simulink model "BE_simu5"  (R2018b)
settings: Solver=VariableStepAuto  StartTime=0.0  StopTime=100  RelTol=1e-3
values from neighbouring files (symbols this model uses):
  assist = 2    [BE_eletr.m]
  lambm = 0.0744    [BE_eletr.m]
  Ls = 0.0021    [BE_eletr.m]
  Np = 52    [BE_eletr.m]
  Rs = 0.124    [BE_eletr.m]
  s = 0.07    [BE_eletr.m]
libraries: simulink x2
settings Model: Creator=antoi  LastModifiedBy=piffercg
settings SolverCC: AlgebraicLoopSolver=LineSearch
settings DataIOCC: ReturnWorkspaceOutputs=on

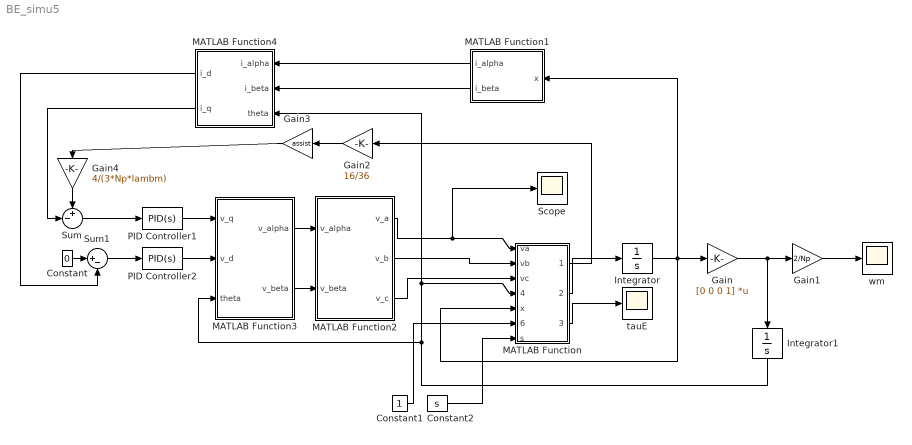
== system BE_simu5 ==
  Constant : Constant  Value=0
  Constant1 : Constant
  Constant2 : Constant  Value=s
  Gain : Gain  Gain=[0 0 0 1]  Multiplication=Matrix(K*u)
  Gain1 : Gain  Gain=2/Np
  Gain2 : Gain  Gain=16/36
  Gain3 : Gain  Gain=assist
  Gain4 : Gain  Gain=4/(3*Np*lambm)
  Integrator : Integrator  InitialCondition=[0 ;0 ;0;0]
  Integrator1 : Integrator
  MATLAB Function : MATLAB Function  TreatAsAtomicUnit=on
  MATLAB Function1 : MATLAB Function  TreatAsAtomicUnit=on
  MATLAB Function2 : MATLAB Function  TreatAsAtomicUnit=on
  MATLAB Function3 : MATLAB Function  TreatAsAtomicUnit=on
  MATLAB Function4 : MATLAB Function  TreatAsAtomicUnit=on
  PID Controller1 : simulink/Continuous/PID Controller  Controller=PID  Form=Parallel  TimeDomain=Continuous-time  SampleTime=-1  IntegratorMethod=Forward Euler  FilterMethod=Forward Euler  ControllerParametersSource=internal  P=Rs  I=Rs*Rs/Ls  D=0  UseFilter=on  N=100  TunerSelectOption=Transfer Function Based (PID Tuner App)  InitialConditionSource=internal  InitialConditionForIntegrator=0  InitialConditionForFilter=0  DifferentiatorICPrevScaledInput=0  ExternalReset=none  TrackingMode=off  Kt=1  LimitOutput=off  UpperSaturationLimit=inf  LowerSaturationLimit=-inf  LinearizeAsGain=on  AntiWindupMode=none  Kb=1  POutMin=[]  POutMax=[]  IOutMin=[]  IOutMax=[]  DOutMin=[]  DOutMax=[]  NOutMin=[]  NOutMax=[]  SumOutMin=[]  SumOutMax=[]  SaturationOutMin=[]  SaturationOutMax=[]  PParamMin=[]  PParamMax=[]  IParamMin=[]  IParamMax=[]  DParamMin=[]  DParamMax=[]  NParamMin=[]  NParamMax=[]  KbParamMin=[]  KbParamMax=[]  KtParamMin=[]  KtParamMax=[]  KbOutMin=[]  KbOutMax=[]  KtOutMin=[]  KtOutMax=[]  IntegratorOutMin=[]  IntegratorOutMax=[]  FilterOutMin=[]  FilterOutMax=[]  SumI1OutMin=[]  SumI1OutMax=[]  SumI2OutMin=[]  SumI2OutMax=[]  SumI3OutMin=[]  SumI3OutMax=[]  SumI4OutMin=[]  SumI4OutMax=[]  SumDOutMin=[]  SumDOutMax=[]  DifferentiatorOutMin=[]  DifferentiatorOutMax=[]  FilterDiffOutCoefMin=[]  FilterDiffOutCoefMax=[]  ReciprocalOutMin=[]  ReciprocalOutMax=[]  SumDenOutMin=[]  SumDenOutMax=[]  SumNumOutMin=[]  SumNumOutMax=[]  DivideOutMin=[]  DivideOutMax=[]  IntegratorContinuousStateAttributes=''  IntegratorStateMustResolveToSignalObject=off  IntegratorRTWStateStorageClass=Auto  FilterContinuousStateAttributes=''  FilterStateMustResolveToSignalObject=off  FilterRTWStateStorageClass=Auto  ParallelPVariant=InternalParameters  IdealPVariant=Disabled  IVariant=InternalParameters  DVariant=InternalParameters  IntegratorVariant=Continuous  SatVariant=Disabled  AWVariant=Passthrough  PCopyVariant=Disabled  TRVariant=Disabled  FdbkBlocksVariant=Forward  IdealPFdbkVariant=Disabled  SatFdbkVariant=Disabled  DerivativeFilterVariant=ContFilter  NVariant=InternalParameters  NCopyVariant=Disabled  FilterICVariant=InternalICsFilter  IntegratorICVariant=InternalICs  ExternalResetVariant=Disabled  TRSumVariant=Passthrough  SumFdbkVariant=Disabled  SumVariant=Sum_PID
  PID Controller2 : simulink/Continuous/PID Controller  Controller=PID  Form=Parallel  TimeDomain=Continuous-time  SampleTime=-1  IntegratorMethod=Forward Euler  FilterMethod=Forward Euler  ControllerParametersSource=internal  P=Rs  I=Rs*Rs/Ls  D=0  UseFilter=on  N=100  TunerSelectOption=Transfer Function Based (PID Tuner App)  InitialConditionSource=internal  InitialConditionForIntegrator=0  InitialConditionForFilter=0  DifferentiatorICPrevScaledInput=0  ExternalReset=none  TrackingMode=off  Kt=1  LimitOutput=off  UpperSaturationLimit=inf  LowerSaturationLimit=-inf  LinearizeAsGain=on  AntiWindupMode=none  Kb=1  POutMin=[]  POutMax=[]  IOutMin=[]  IOutMax=[]  DOutMin=[]  DOutMax=[]  NOutMin=[]  NOutMax=[]  SumOutMin=[]  SumOutMax=[]  SaturationOutMin=[]  SaturationOutMax=[]  PParamMin=[]  PParamMax=[]  IParamMin=[]  IParamMax=[]  DParamMin=[]  DParamMax=[]  NParamMin=[]  NParamMax=[]  KbParamMin=[]  KbParamMax=[]  KtParamMin=[]  KtParamMax=[]  KbOutMin=[]  KbOutMax=[]  KtOutMin=[]  KtOutMax=[]  IntegratorOutMin=[]  IntegratorOutMax=[]  FilterOutMin=[]  FilterOutMax=[]  SumI1OutMin=[]  SumI1OutMax=[]  SumI2OutMin=[]  SumI2OutMax=[]  SumI3OutMin=[]  SumI3OutMax=[]  SumI4OutMin=[]  SumI4OutMax=[]  SumDOutMin=[]  SumDOutMax=[]  DifferentiatorOutMin=[]  DifferentiatorOutMax=[]  FilterDiffOutCoefMin=[]  FilterDiffOutCoefMax=[]  ReciprocalOutMin=[]  ReciprocalOutMax=[]  SumDenOutMin=[]  SumDenOutMax=[]  SumNumOutMin=[]  SumNumOutMax=[]  DivideOutMin=[]  DivideOutMax=[]  IntegratorContinuousStateAttributes=''  IntegratorStateMustResolveToSignalObject=off  IntegratorRTWStateStorageClass=Auto  FilterContinuousStateAttributes=''  FilterStateMustResolveToSignalObject=off  FilterRTWStateStorageClass=Auto  ParallelPVariant=InternalParameters  IdealPVariant=Disabled  IVariant=InternalParameters  DVariant=InternalParameters  IntegratorVariant=Continuous  SatVariant=Disabled  AWVariant=Passthrough  PCopyVariant=Disabled  TRVariant=Disabled  FdbkBlocksVariant=Forward  IdealPFdbkVariant=Disabled  SatFdbkVariant=Disabled  DerivativeFilterVariant=ContFilter  NVariant=InternalParameters  NCopyVariant=Disabled  FilterICVariant=InternalICsFilter  IntegratorICVariant=InternalICs  ExternalResetVariant=Disabled  TRSumVariant=Passthrough  SumFdbkVariant=Disabled  SumVariant=Sum_PID
  Scope : Scope
  Sum : Sum  Inputs=+-|
  Sum1 : Sum  Inputs=|+-
  tauE : Scope
  wm : Scope
  wires:
  MATLAB Function3/2(v_beta) -> MATLAB Function2/2(v_beta)
  MATLAB Function3/1(v_alpha) -> MATLAB Function2/1(v_alpha)
  Integrator/1 -> MATLAB Function1/1(x), MATLAB Function/5(x), Gain/1
  Gain/1 -> Integrator1/1, Gain1/1
  Integrator1/1 -> MATLAB Function/4(thetaE), MATLAB Function4/3(theta), MATLAB Function3/3(theta)
  MATLAB Function/3(tauE) -> tauE/1
  MATLAB Function/2(xdot) -> Integrator/1
  MATLAB Function2/1(v_a) -> Scope/1, MATLAB Function/1(va)
  Constant2/1 -> MATLAB Function/7(s)
  Constant1/1 -> MATLAB Function/6(pedaling)
  Sum/1 -> PID Controller1/1
  Gain2/1 -> Gain3/1
  MATLAB Function/1(tauC) -> Gain2/1
  MATLAB Function1/2(i_beta) -> MATLAB Function4/2(i_beta)
  MATLAB Function1/1(i_alpha) -> MATLAB Function4/1(i_alpha)
  Sum1/1 -> PID Controller2/1
  Constant/1 -> Sum1/1
  MATLAB Function4/1(i_d) -> Sum1/2
  MATLAB Function4/2(i_q) -> Sum/2
  Gain1/1 -> wm/1
  Gain4/1 -> Sum/1
  Gain3/1 -> Gain4/1
  PID Controller1/1 -> MATLAB Function3/1(v_q)
  PID Controller2/1 -> MATLAB Function3/2(v_d)
  MATLAB Function2/2(v_b) -> MATLAB Function/2(vb)
  MATLAB Function2/3(v_c) -> MATLAB Function/3(vc)

== matlab function BE_simu5/MATLAB Function1 ==
  data: x input; i_alpha output; i_beta output
function [i_alpha, i_beta] = Clarke(x)
i_alpha = x(1);
i_beta = (x(1)+2*x(2))/sqrt(3);
end

== matlab function BE_simu5/MATLAB Function ==
  data: tauC output; va input; vb input; vc input; xdot output; thetaE input; x input; tauE output; pedaling input; s input
function [tauC,xdot,tauE] = fcn(va,vb,vc,thetaE,x, pedaling,s)
Rs = 0.124 ;
Ls = 0.0021 ;
Lambdam = 0.0744 ;
Np = 52 ;
M = 92 ;
Rw = 0.33 ;
Jt = M*Rw*Rw ;
Ca = 0.18 ;
g = 9.81 ;
tauE = (Np/2)*(x(1)*Lambdam*(-sin(thetaE))+x(2)*Lambdam*(-sin(thetaE-2*pi/3))+x(3)*Lambdam*(-sin(thetaE+2*pi/3)));
tauC = (60 - (60/(4*pi))*x(4)*(16/36)*(2/Np))*pedaling ; 
tauload = M*g*s*Rw + Ca*Rw*Rw*Rw*x(4)*x(4)*(4/(Np*Np)) ;
xdot1 = va/Ls - (Rs/Ls)*x(1) + (Lambdam/Ls)*x(4)*sin(thetaE) ; 
xdot2 = vb/Ls - (Rs/Ls)*x(2) + (Lambdam/Ls)*x(4)*sin(thetaE -2*pi/3) ;
xdot3 = vc/Ls - (Rs/Ls)*x(3) + (Lambdam/Ls)*x(4)*sin(thetaE +2*pi/3) ;
xdot4 = (Np/(2*Jt))*(tauE - tauload + tauC*16/36)  ;
xdot=[xdot1;xdot2;xdot3;xdot4] ;
end

== matlab function BE_simu5/MATLAB Function2 ==
  data: v_alpha input; v_a output; v_beta input; v_b output; v_c output
function [v_a, v_b,v_c] = inv_Clarke(v_alpha,v_beta)
v_a = v_alpha ;
v_b = -v_alpha/2 + sqrt(3)*v_beta/2 ;
v_c = -v_a-v_b ;
end

== matlab function BE_simu5/MATLAB Function3 ==
  data: v_q input; v_d input; v_alpha output; theta input; v_beta output
function [v_alpha,v_beta] = inv_Park(v_q,v_d,theta)
v_alpha = v_d*cos(theta) - v_q*sin(theta) ; 
v_beta = v_q*cos(theta) + v_d*sin(theta) ;
end

== matlab function BE_simu5/MATLAB Function4 ==
  data: i_alpha input; i_d output; i_beta input; theta input; i_q output
function [i_d,i_q] = Park(i_alpha,i_beta,theta)
i_d = i_alpha*cos(theta)+i_beta*sin(theta);
i_q = -i_alpha*sin(theta)+i_beta*cos(theta);
end
